simulink model "Multiplexing"  (R2024a)
settings: Solver=VariableStepAuto  StartTime=0.0  StopTime=10.0  RelTol=1e-3
libraries: dspfdesign x2
settings Model: Creator=mohamed
settings SolverCC: AlgebraicLoopSolver=TrustRegion
settings DebuggingCC: UnconnectedInputMsg=warning  UnconnectedOutputMsg=warning  UnconnectedLineMsg=warning
settings ModelReferenceCC: EnableRefExpFcnMdlSchedulingChecks=on
settings SFSimCC: CustomCodeUndefinedFunction=UseInterfaceOnly
settings RTWCC: GPUComputeCapability=3.5  DLArmComputeVersion=19.05

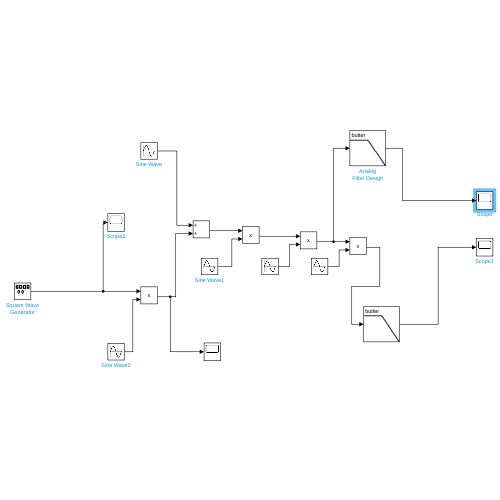
[thumbnail: Simulink's stored preview of the top-level diagram]
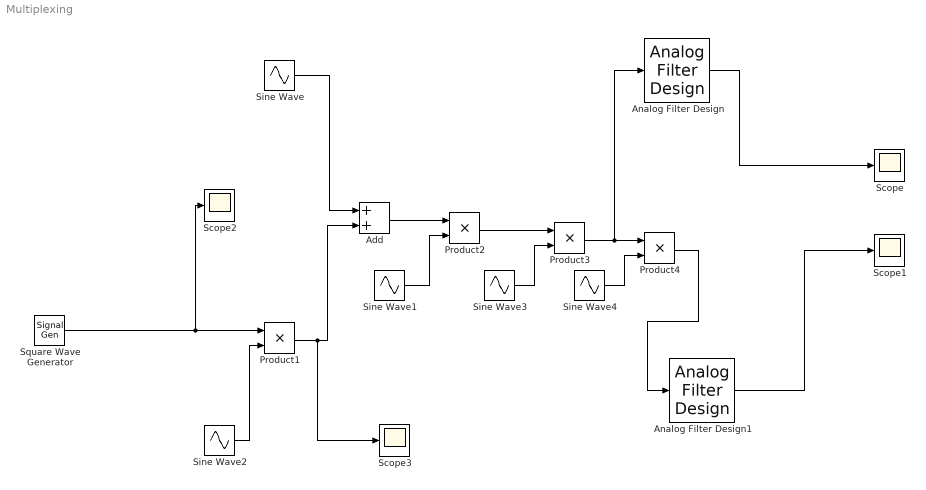
== system Multiplexing ==
  Add : Sum
  Analog Filter Design : dspfdesign/Analog Filter Design  method=Butterworth  filttype=Lowpass  N=8  Wlo=2*pi  Whi=80  Rp=2  Rs=40
  Analog Filter Design1 : dspfdesign/Analog Filter Design  method=Butterworth  filttype=Lowpass  N=8  Wlo=2*4*pi  Whi=80  Rp=2  Rs=40
  Product{1..4} (4 alike) : Product
  Scope{,1..3} (4 alike) : Scope
  Sine Wave : Sin  Frequency=2*pi  SampleTime=0
  Sine Wave1 : Sin  Frequency=2*1000*pi  Phase=pi/2  SampleTime=0
  Sine Wave2 : Sin  Frequency=2*4*pi  Phase=pi/2  SampleTime=0
  Sine Wave3 : Sin  Amplitude=2  Frequency=2*1000*pi  Phase=pi/2  SampleTime=0
  Sine Wave4 : Sin  Frequency=2*4*pi  Phase=pi/2  SampleTime=0
  Square Wave Generator : SignalGenerator  WaveForm=square
  wires:
  Sine Wave/1 -> Add/1
  Sine Wave2/1 -> Product1/2
  Square Wave Generator/1 -> Scope2/1, Product1/1
  Product1/1 -> Scope3/1, Add/2
  Add/1 -> Product2/1
  Sine Wave1/1 -> Product2/2
  Product2/1 -> Product3/1
  Sine Wave3/1 -> Product3/2
  Product3/1 -> Product4/1, Analog Filter Design/1
  Analog Filter Design/1 -> Scope/1
  Sine Wave4/1 -> Product4/2
  Product4/1 -> Analog Filter Design1/1
  Analog Filter Design1/1 -> Scope1/1
